simulink model "rigid_launcher_CL"  (R2020b)
settings: Solver=ode23s  StartTime=0.0  StopTime=100  FixedStep=0.05  RelTol=1e-3  EnableMultiTasking=on
undefined symbols (not defined in the file or in its folder): ak, Ar, betafz, bk, Br, ck, Cr, deltaW, dk, Dr, t0, thetac, ventonoff
settings Model: ExtModeAutoUpdateStatusClock=off  Creator=chiappa  LastModifiedBy=X000274
settings DataIOCC: LimitDataPoints=on  SaveFormat=Array  SignalLoggingSaveFormat=ModelDataLogs  ReturnWorkspaceOutputs=off  SignalLoggingName=sigsOut
settings OptimizationCC: BlockReduction=off  BooleanDataType=off
settings DebuggingCC: SaveWithParameterizedLinksMsg=none  UnderspecifiedInitializationDetection=Classic  MergeDetectMultiDrivingBlocksExec=none  SignalResolutionControl=TryResolveAllWithWarning  MultiTaskDSMMsg=warning  MultiTaskCondExecSysMsg=none  ArithmeticOperatorsInVariantConditions=warning
settings HardwareCC: ProdBitPerPointer=32  ProdBitPerSizeT=32  ProdBitPerPtrDiffT=32  ProdLargestAtomicFloat=None  ProdIntDivRoundTo=Undefined  ProdEndianess=Unspecified  ProdWordSize=32  ProdHWDeviceType=32-bit Generic  TargetUnknown=on
settings ModelReferenceCC: PropagateSignalLabelsOutOfModel=off
settings SFSimCC: SimUseLocalCustomCode=off  CustomCodeUndefinedFunction=UseInterfaceOnly
settings RTWCC: RTWUseLocalCustomCode=off
settings GRTTargetCC: TargetLangStandard=C89/C90 (ANSI)  CombineOutputUpdateFcns=off  GRTInterface=on
settings ConfigComp: CovMetricSettings=dw  CovSaveCumulativeToWorkspaceVar=on  CovSaveSingleToWorkspaceVar=on  CovExternalEMLEnable=off

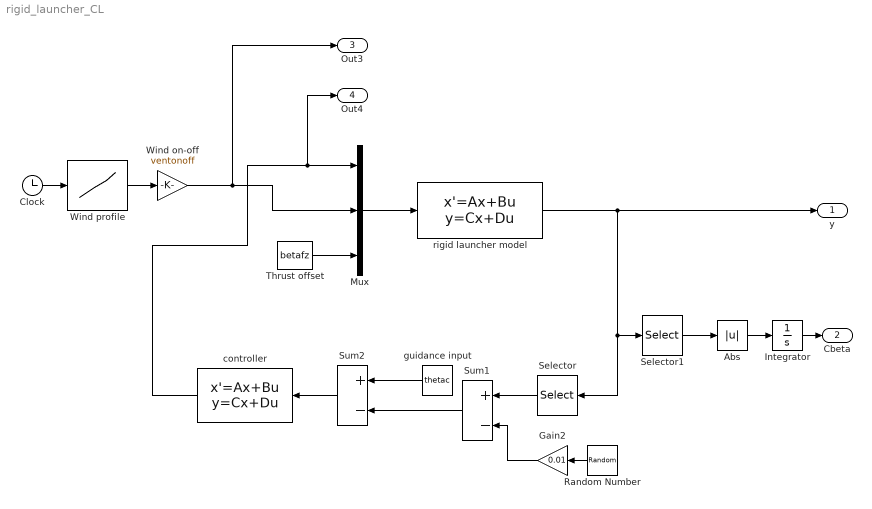
== system rigid_launcher_CL ==
  Abs : Abs
  Clock : Clock
      settings: Decimation=100
  Gain2 : Gain  Gain=0.01  SaturateOnIntegerOverflow=on  OutDataTypeStr=Inherit: Same as input  ParamDataTypeStr=Inherit: Same as input
  Integrator : Integrator
  Mux : Mux  Inputs=3
  Random Number : RandomNumber  Variance=0.022*3.14/180  SampleTime=0.1
  Selector : Selector  InputPortWidth=6  IndexOptions=Index vector (dialog)  Indices=[2]  OutputSizes=1
  Selector1 : Selector  InputPortWidth=6  IndexOptions=Index vector (dialog)  Indices=[4]  OutputSizes=1
  Sum1 : Sum  Inputs=+-  InputSameDT=on  SaturateOnIntegerOverflow=on  OutDataTypeStr=Inherit: Same as first input
  Sum2 : Sum  Inputs=+-  InputSameDT=on  SaturateOnIntegerOverflow=on  OutDataTypeStr=Inherit: Same as first input
  Thrust offset : Constant  Value=betafz
  Wind on-off : Gain  Gain=ventonoff  SaturateOnIntegerOverflow=on  OutDataTypeStr=Inherit: Same as input  ParamDataTypeStr=Inherit: Same as input
  Wind profile : Lookup  InputValues=t0  Table=deltaW  SaturateOnIntegerOverflow=on
  controller : StateSpace  A=ak  B=bk  C=ck  D=dk  InitialCondition=0
  guidance input : Constant  Value=thetac
  rigid launcher model : StateSpace  A=Ar  B=Br  C=Cr  D=Dr  InitialCondition=0
  y : Outport  VectorParamsAs1DForOutWhenUnconnected=off
  Cbeta : Outport  Port=2  VectorParamsAs1DForOutWhenUnconnected=off
  Out3 : Outport  Port=3  VectorParamsAs1DForOutWhenUnconnected=off
  Out4 : Outport  Port=4  VectorParamsAs1DForOutWhenUnconnected=off
  wires:
  Mux/1 -> rigid launcher model/1
  rigid launcher model/1 -> y/1, Selector/1, Selector1/1
  Clock/1 -> Wind profile/1
  Wind profile/1 -> Wind on-off/1
  Selector1/1 -> Abs/1
  Abs/1 -> Integrator/1
  Thrust offset/1 -> Mux/3
  Integrator/1 -> Cbeta/1
  Selector/1 -> Sum1/1
  Random Number/1 -> Gain2/1
  Gain2/1 -> Sum1/2
  Wind on-off/1 -> Mux/2, Out3/1
  Sum1/1 -> Sum2/2
  Sum2/1 -> controller/1
  guidance input/1 -> Sum2/1
  controller/1 -> Mux/1, Out4/1
